simulink model "especies"  (R2021b)
settings: Solver=VariableStepAuto  StartTime=0.0  StopTime=500  FixedStep=0.938813135927453  RelTol=1e-3
model workspace (MAT data in the model file):
  a = 0.2586
  b = 0.0203
  c = 0.0574
  d = 0.00975
  m = 0.0571
  n = 0.0048
  x0 = 0.4184
  y0 = 0.6315
settings Model: Creator=LuisaToro  LastModifiedBy=LuisaToro
settings DataIOCC: SaveFormat=Array  OutputTimes=tout

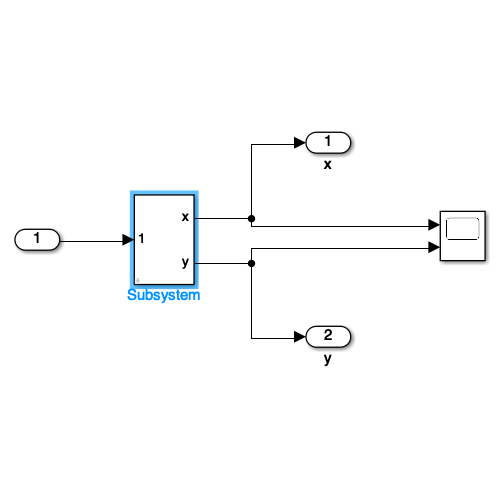
[thumbnail: Simulink's stored preview of the top-level diagram]
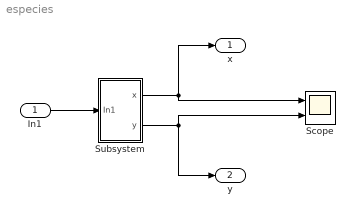
== system especies ==
  In1 : Inport  OutMin=-1  OutMax=0
  Scope : Scope  NumInputPorts=2
  Subsystem : Subsystem  mask{a=a, b=b, c=c, d=d, m=m, n=n, x0=x0, y0=y0}
  x : Outport
  y : Outport  Port=2
  wires:
  Subsystem/1(x) -> Scope/1, x/1
  Subsystem/2(y) -> y/1, Scope/2
  In1/1 -> Subsystem/1(In1)

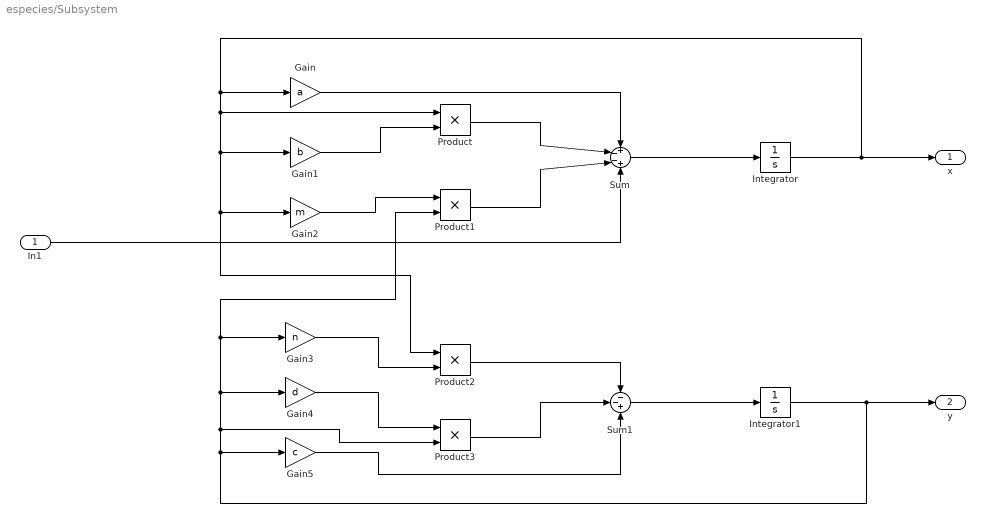
== system especies/Subsystem ==
  In1 : Inport
  Gain : Gain  Gain=a
  Gain1 : Gain  Gain=b
  Gain2 : Gain  Gain=m
  Gain3 : Gain  Gain=n
  Gain4 : Gain  Gain=d
  Gain5 : Gain  Gain=c
  Integrator : Integrator  InitialCondition=x0
  Integrator1 : Integrator  InitialCondition=y0
  Product{,1..3} (4 alike) : Product
  Sum : Sum  Inputs=+--+
  Sum1 : Sum  Inputs=--+
  x : Outport
  y : Outport  Port=2
  wires:
  Product2/1 -> Sum1/1
  Gain/1 -> Sum/1
  Product1/1 -> Sum/3
  Gain1/1 -> Product/2
  Product3/1 -> Sum1/2
  Sum1/1 -> Integrator1/1
  Gain3/1 -> Product2/2
  Product/1 -> Sum/2
  Integrator/1 -> x/1, Product/1, Product2/1, Gain2/1, Gain1/1, Gain/1
  Sum/1 -> Integrator/1
  Gain4/1 -> Product3/1
  In1/1 -> Sum/4
  Integrator1/1 -> y/1, Product3/2, Product1/2, Gain3/1, Gain4/1, Gain5/1
  Gain2/1 -> Product1/1
  Gain5/1 -> Sum1/3
